simulink model "AAItest"  (R2020a)
settings: Solver=FixedStepAuto  StartTime=0.0  StopTime=10.0  FixedStep=1e-3  RelTol=1e-3  EnableMultiTasking=on
undefined symbols (not defined in the file): D0, D10, D11, D12, D13, D2, D4, D5, D6, D7, D8, D9, PTA0, PTA2, PTB23, PTB9, PTC16, PTC2, PTC3, PTC4, PTD0, PTD1, PTD2, PTD3
libraries: frdmk64flib x12
settings Model: ExtModeTrigDuration=5  Creator=rafit  LastModifiedBy=rafit
settings OptimizationCC: EnhancedBackFolding=on  PassReuseOutputArgsAs=Individual arguments  ZeroExternalMemoryAtStartup=off  ZeroInternalMemoryAtStartup=off  MaxStackSize=64  OptimizeBlockOrder=speed  DifferentSizesBufferReuse=on  OptimizationCustomize=off  EfficientTunableParamExpr=on
settings DebuggingCC: ParameterTunabilityLossMsg=error
settings HardwareCC: ProdBitPerPointer=32  ProdBitPerSizeT=32  ProdBitPerPtrDiffT=32  ProdLargestAtomicInteger=Long  ProdLargestAtomicFloat=Double  ProdWordSize=32  ProdHWDeviceType=ARM Compatible->ARM Cortex
settings SFSimCC: MATLABDynamicMemAlloc=off
settings RTWCC: SystemTargetFile=ert.tlc  HardwareBoard=NXP FRDM-K64F  TemplateMakefile=ert_default_tmf  Toolchain=GNU Tools for ARM Embedded Processors
settings CodeAppCC: ForceParamTrailComments=on  IgnoreCustomStorageClasses=off  OperatorAnnotations=on  SimulinkDataObjDesc=on  SFDataObjDesc=on  InsertBlockDesc=on

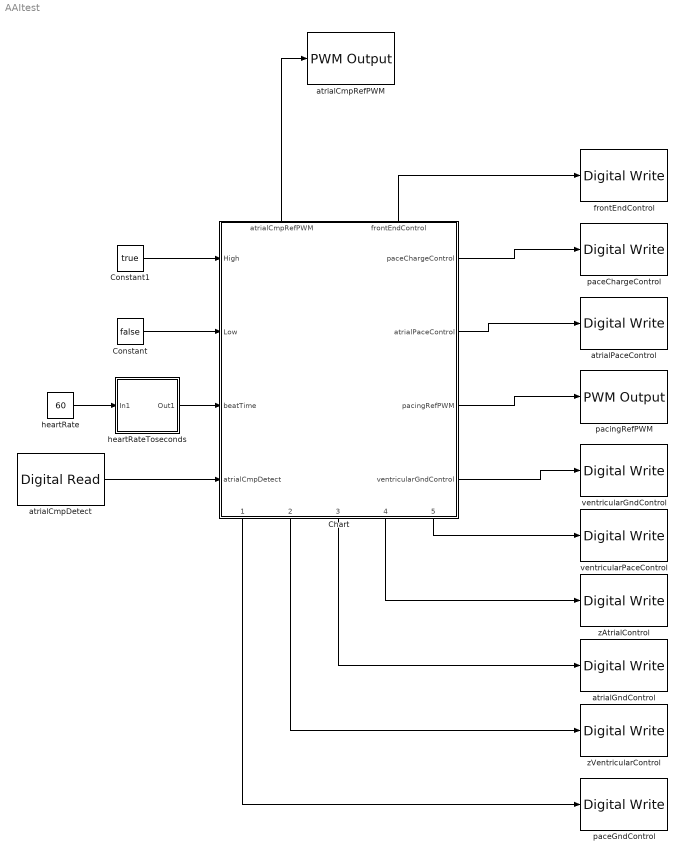
== system AAItest ==
  Chart : Stateflow chart  TreatAsAtomicUnit=on
      settings: PortSchema="{\"entries\":[{\"content\":{\"sides\":[{\"content\":{\"connectorIds\":[\"In1\",\"In2\",\"In3\",\"In4\"]},\"type\":\"ConnectorPlacement.EquallySpacedRectSide\",\"uuid\":\"1030ba94-3d3a-48a3-b1f1-8404633e8ae7\"},{\"content\":{\"connectorIds\":[\"Out6\",\"Out7\",\"Out8\",\"Out9\"],\"side\":\"RIGHT\"},\"type\":\"ConnectorPlacement.EquallySpacedRectSide\",\"uuid\":\"6ea2fafc-3ccc-49f0-b2c6-f7c2ccbcd426\"},{\"content\":{\"connectorIds\":[\"Out11\",\"Out10\"],\"side\":\"TOP\"},\"type\":\"ConnectorPlacement.EquallySpacedRectSide\",\"uuid\":\"aef035b1-dd5c-4412-9139-3b9093403f25\"},{\"content\":{\"connectorIds\":[\"Out1\",\"Out2\",\"Out3\",\"Out4\",\"Out5\"],\"side\":\"BOTTOM\"},\"type\":\"ConnectorPlacement.EquallySpacedRectSide\",\"uuid\":\"e8f47484-6116-43fa-985d-197ca0b53ad8\"}]},\"type\":\"ConnectorPlacement.EquallySpacedConnector\",\"uuid\":\"105d53bb-c734-4637-b038-9b0b6c1e571f\"}],\"packageUris\":[\"http://schema.mathworks.com/mf0/Connector/19700101\"],\"version\":\"1.0\"}"
  Constant : Constant  Value=false
  Constant1 : Constant  Value=true
  atrialCmpDetect : frdmk64flib/Digital Read  Whichpin=PTC16 (D0)  SampleTime=0.001
  atrialCmpRefPWM : frdmk64flib/PWM Output  Whichpin=PTC2 (D6)  InitialFrequency=2000  InitialDutyCycle=0
  atrialGndControl : frdmk64flib/Digital Write  Whichpin=PTD2 (D11)
  atrialPaceControl : frdmk64flib/Digital Write  Whichpin=PTA0 (D8)
  frontEndControl : frdmk64flib/Digital Write  Whichpin=PTD1 (D13)
  heartRate : Constant  Value=60
  heartRateToseconds : Subsystem
  paceChargeControl : frdmk64flib/Digital Write  Whichpin=PTB9 (D2)
  paceGndControl : frdmk64flib/Digital Write  Whichpin=PTD0 (D10)
  pacingRefPWM : frdmk64flib/PWM Output  Whichpin=PTA2 (D5)  InitialFrequency=2000  InitialDutyCycle=0
  ventricularGndControl : frdmk64flib/Digital Write  Whichpin=PTD3 (D12)
  ventricularPaceControl : frdmk64flib/Digital Write  Whichpin=PTC4 (D9)
  zAtrialControl : frdmk64flib/Digital Write  Whichpin=PTB23 (D4)
  zVentricularControl : frdmk64flib/Digital Write  Whichpin=PTC3 (D7)
  wires:
  heartRateToseconds/1(Out1) -> Chart/3(beatTime)
  heartRate/1 -> heartRateToseconds/1(In1)
  Chart/2(zVentricularControl) -> zVentricularControl/1
  Chart/7(atrialPaceControl) -> atrialPaceControl/1
  Chart/4(zAtrialControl) -> zAtrialControl/1
  Chart/3(atrialGndControl) -> atrialGndControl/1
  Constant1/1 -> Chart/1(High)
  Chart/1(paceGndControl) -> paceGndControl/1
  Chart/9(ventricularGndControl) -> ventricularGndControl/1
  Chart/5(ventricularPaceControl) -> ventricularPaceControl/1
  Chart/6(paceChargeControl) -> paceChargeControl/1
  Constant/1 -> Chart/2(Low)
  Chart/8(pacingRefPWM) -> pacingRefPWM/1
  Chart/11(atrialCmpRefPWM) -> atrialCmpRefPWM/1
  Chart/10(frontEndControl) -> frontEndControl/1
  atrialCmpDetect/1 -> Chart/4(atrialCmpDetect)

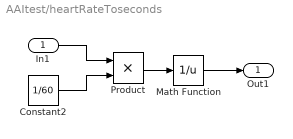
== system AAItest/heartRateToseconds ==
  In1 : Inport
  Constant2 : Constant  Value=1/60
  Math Function : Math  Operator=reciprocal  SaturateOnIntegerOverflow=on
  Product : Product
  Out1 : Outport
  wires:
  Product/1 -> Math Function/1
  Constant2/1 -> Product/2
  In1/1 -> Product/1
  Math Function/1 -> Out1/1

== stateflow chart AAItest/Chart ==
  state dischargeBlocking
    entry:
    pacingRefPWM = 0;
    paceChargeControl = Low;
    %changesBelow
    paceGndControl = High;
    ventricularPaceControl = Low;
    zAtrialControl = Low;
    zVentricularControl = Low;
    atrialPaceControl = Low;
    atrialGndControl = High;
    ventricularGndControl = Low;
  state senseSignal
    entry:
    signalDetected = Low;
    frontEndControl = High;
    atrialCmpRefPWM = 90;
    during:
    signalDetected = atrialCmpDetect;
  state discharging
    entry:
    pacingRefPWM = 0;
    paceChargeControl = Low;
    paceGndControl = High;
    atrialPaceControl = High;
    atrialGndControl = Low;
    zAtrialControl = Low;
    zVentricularControl = Low;
    ventricularGndControl = Low;
    ventricularPaceControl = Low;
  state charging
    entry:
    atrialPaceControl = Low;
    ventricularPaceControl = Low;
    pacingRefPWM = 100;
    paceChargeControl = High;
    paceGndControl = Low;
    atrialGndControl = Low;
    zAtrialControl = Low;
    zVentricularControl = Low;
    ventricularGndControl = Low;
  (default) -> senseSignal
  dischargeBlocking -> senseSignal : [after(1,msec)]
  senseSignal -> senseSignal [order 1] : [atrialCmpDetect == High]
  senseSignal -> charging [order 2] : [after(beatTime,sec)]
  discharging -> dischargeBlocking : [after(1,msec)]
  charging -> discharging : [after(10,msec)]
  data: High input; paceGndControl output; zVentricularControl output; atrialGndControl output; zAtrialControl output; ventricularPaceControl output; paceChargeControl output; atrialPaceControl output; pacingRefPWM output; ventricularGndControl output; Low input; beatTime input; signalDetected local; frontEndControl output; atrialCmpRefPWM output; atrialCmpDetect input
